simulink model "EVdemo_6"  (R2013b)
settings: Solver=FixedStepDiscrete  SolverMode=SingleTasking  StartTime=0.0  StopTime=650  FixedStep=4e-5  MaxStep=1e-5  RelTol=1e-3
InitFcn:
  | %EV_Param_Update
  | % update the number of strings (discretized)
  | numStrings = round(Opti_numStrings);
  | %disp(['Number of strings: ' num2str(numStrings)])
  | % update the effective capacity based on the number of strings
  | EV_Param.Battery_Det.Rated_Capacity = 28.5*numStrings; %A*hr
  | EV_Param.Battery_Det.DP = 1.5*fliplr([1500 1500 1600 1450 1325 1125 925 675 425 175 ])./8*EV_Param.Battery_Det.Rated_Capacity; % 8 comes from the 8Ahr rated batter data used (normalize and rescale to the rated capacity
  | EV_Param.Battery_Det.CP = fliplr([25 100 200 250 375 550 750 950 1125 1150])./8*EV_Param.Battery_Det.Rated_Capacity;
  | 
  | % update the number of cells in a string (discretized)
  | numSeriesCells = round(Opti_numSeriesCells);
  | %disp(['Number of cells in a string: ' num2str(numSeriesCells)])
  | % update the nominal string volage and charge deficit
  | EV_Param.Battery_Det.Nominal_Voltage = numSeriesCells*cellVolts;
  | BatteryParams(1).Qe_init = 0;%EV_Param.Battery_Det.Rated_Capacity*(1-EV_Param.Battery_Det.Initial_SOC/100); %Ampere*hours
  | 
  | % update the total number of cells, battery pack mass and total vehicle
  | % mass
  | total_cells = numSeriesCells*numStrings;
  | %disp(['Total Number of cells: ' num2str(total_cells)])
  | EV_Param.BatteryMass = BatteryParams(1).cell_mass*total_cells;
  | %disp(['Total Battery Pack Mass: ' num2str(EV_Param.BatteryMass)])
  | EV_Param.Vehicle.Mass = 1300+EV_Param.BatteryMass;
  | 
  | % update the driveline gear ratio
  | EV_Param.Vehicle.Engine_Vehicle_Gear_Ratio = Opti_Vehicle_Gear_Ratio;
  | %disp(['Driveline gear ratio: ' num2str(Opti_Vehicle_Gear_Ratio)])
StartFcn:
  | %tic;
StopFcn:
  | %toc;
  | %disp([Final SOC: ' num2str(SOC_final)])
  | %disp([Final Vehicle Error: ' num2str(normed_SQE_final)])
model workspace (MAT data in the model file):
  MCOS : class17 (value not decoded)
  MCOS : class17 (value not decoded)
values from neighbouring files (symbols this model uses):
  Drive_Cycle_Num = 8    [startDemo.m]
undefined symbols (not defined in the file or in its folder): Acc_Cmd, BatteryParams, Brake_Set, cell_area, ctrlConst, current_phase_a, Dec_Cmd, direct_current, DiscIntNeverNeededParam, electromagnetic_torque, HEV_Param, Ion, Kt_Temps, Lithium, Mech_Power_kW, Opti_numSeriesCells, Opti_numStrings, Opti_Vehicle_Gear_Ratio, paramVelocityI, paramVelocityP, paramVelocityPICurrentSat, pmsm, quadrature_current, RLoadLoss, rotor_velocity, sigbuilder_block, Ts, Veh_Spd_Ref
libraries: fl_lib x306, nesl_utility x100, LeadAcidBattery_lib x60, simulink x23, powerlib x16, sdl_lib x7, elec_lib x4, electricdrivelib x2, checkpacklib x2, CustomDriveline_lib x2, LiBatteryBlocks x1, Capacitors_lib x1
(part 5 of 7)

== system EVdemo_6/Battery/Cells/Battery cell8 ==
  C1 : LeadAcidBattery_lib/Main Branch Capacitance, C1  Tau1=HEV_Param.Battery_Cell.Tau1 s  Cmin=1e-5 F  i_Log=off  Q_Log=off  LocalVarNames=|i|v|Q  LocalVarDescs=|Current through variable|Voltage across variable|Charge variable  LocalVarLogging=[0 0 0]
  Diode : fl_lib/Electrical/Electrical Elements/Diode  Vf=0.6 V  Ron=0.3 Ohm  Goff=1e-08 1/Ohm  i_Log=off  v_Log=off  LocalVarNames=|current|voltage|power  LocalVarDescs=|Diode current (A)|Voltage across diode (V)|Power (W)  LocalVarLogging=[0 0 0]
  Ep : fl_lib/Electrical/Electrical Sources/DC Voltage Source  v0=HEV_Param.Battery_Cell.Ep V  i_Log=off  v_Log=off  LocalVarNames=|current|voltage|power  LocalVarDescs=|Current (A)|Voltage (V)|Power (W)  LocalVarLogging=[0 0 0]
  Main Branch Voltage Source (Em) : LeadAcidBattery_lib/Main Branch Voltage Source, Em  Em0=HEV_Param.Battery_Cell.Emo V  Ke=HEV_Param.Battery_Cell.Ke V/K  Kc=HEV_Param.Battery_Cell.Kc  C0=HEV_Param.Battery_Cell.Costar s*A  Istar=HEV_Param.Battery_Cell.Istar A  delta=HEV_Param.Battery_Cell.delta  Tau1=HEV_Param.Battery_Cell.Tau1 s  Qinit=HEV_Param.Battery_Cell.Qe_init s*A  i_Log=off  Iavg_Log=off  Qe_Log=off  LocalVarNames=|i|v|cap_u|cap_t|Q|Iavg  LocalVarDescs=|Current through variable|Voltage across variable|usable battery capacity|total battery capacity|battery charge|average current given by (I/(Ts+1))  LocalVarLogging=[0 0 0 0 0 0]
  R0 : LeadAcidBattery_lib/Terminal Resistance, R0  R00=HEV_Param.Battery_Cell.Roo Ohm  A0=HEV_Param.Battery_Cell.Ao  i_Log=off  LocalVarNames=|i|v  LocalVarDescs=|Current through variable|Voltage across variable  LocalVarLogging=[0 0]
  R1 : LeadAcidBattery_lib/Main Branch Resistance, R1  R10=HEV_Param.Battery_Cell.R10 Ohm  DOC_min=1e-006  i_Log=off  LocalVarNames=|i|v  LocalVarDescs=|Current through variable|Voltage across variable  LocalVarLogging=[0 0]
  R2 : LeadAcidBattery_lib/Main Branch Resistance, R2  R20=HEV_Param.Battery_Cell.R20 Ohm  A21=HEV_Param.Battery_Cell.A21  A22=HEV_Param.Battery_Cell.A22  Istar=HEV_Param.Battery_Cell.Istar A  i_Log=off  LocalVarNames=|i|v  LocalVarDescs=|Current through variable|Voltage across variable  LocalVarLogging=[0 0]
  Rp : LeadAcidBattery_lib/Parasitic Branch Resistance, Rp  Gp0=HEV_Param.Battery_Cell.Gpo 1/Ohm  Vp0=HEV_Param.Battery_Cell.Vpo V  Ap=HEV_Param.Battery_Cell.Ap  Tf=HEV_Param.Battery_Cell.theta_f C  i_Log=off  LocalVarNames=|i|v|Vavg  LocalVarDescs=|Current through variable|Voltage across variable|average voltage given by (V/(Ts+1))  LocalVarLogging=[0 0 0]
  Thermal Model : Subsystem
  H : PMIOPort  Tag=PMCPort  Port=1  Side=Left
  + : PMIOPort  Tag=PMCPort  Port=2  Side=Left
  - : PMIOPort  Tag=PMCPort  Port=3  Side=Right
  connections:
  Diode/LConn1 -- R0/RConn1 -- R2/LConn2
  R2/RConn2 -- Thermal Model/LConn1
  -/RConn1 -- Ep/RConn1 -- Main Branch Voltage Source (Em)/RConn1
  Thermal Model/RConn1 -- Main Branch Voltage Source (Em)/RConn3
  Diode/RConn1 -- Rp/LConn1
  Ep/LConn1 -- Rp/RConn2
  Thermal Model/LConn2 -- H/RConn1
  R0/LConn1 -- R2/LConn1 -- Main Branch Voltage Source (Em)/LConn1
  R1/LConn2 -- C1/LConn1
  R1/LConn1 -- C1/LConn2 -- R2/RConn1
  Main Branch Voltage Source (Em)/LConn3 -- C1/RConn1 -- R1/RConn2
  R1/RConn1 -- Main Branch Voltage Source (Em)/LConn2
  R0/LConn2 -- +/RConn1
  Thermal Model/RConn2 -- Main Branch Voltage Source (Em)/RConn2 -- Rp/RConn1

== system EVdemo_6/Battery/Cells/Battery cell9 ==
  C1 : LeadAcidBattery_lib/Main Branch Capacitance, C1  Tau1=HEV_Param.Battery_Cell.Tau1 s  Cmin=1e-5 F  i_Log=off  Q_Log=off  LocalVarNames=|i|v|Q  LocalVarDescs=|Current through variable|Voltage across variable|Charge variable  LocalVarLogging=[0 0 0]
  Diode : fl_lib/Electrical/Electrical Elements/Diode  Vf=0.6 V  Ron=0.3 Ohm  Goff=1e-08 1/Ohm  i_Log=off  v_Log=off  LocalVarNames=|current|voltage|power  LocalVarDescs=|Diode current (A)|Voltage across diode (V)|Power (W)  LocalVarLogging=[0 0 0]
  Ep : fl_lib/Electrical/Electrical Sources/DC Voltage Source  v0=HEV_Param.Battery_Cell.Ep V  i_Log=off  v_Log=off  LocalVarNames=|current|voltage|power  LocalVarDescs=|Current (A)|Voltage (V)|Power (W)  LocalVarLogging=[0 0 0]
  Main Branch Voltage Source (Em) : LeadAcidBattery_lib/Main Branch Voltage Source, Em  Em0=HEV_Param.Battery_Cell.Emo V  Ke=HEV_Param.Battery_Cell.Ke V/K  Kc=HEV_Param.Battery_Cell.Kc  C0=HEV_Param.Battery_Cell.Costar s*A  Istar=HEV_Param.Battery_Cell.Istar A  delta=HEV_Param.Battery_Cell.delta  Tau1=HEV_Param.Battery_Cell.Tau1 s  Qinit=HEV_Param.Battery_Cell.Qe_init s*A  i_Log=off  Iavg_Log=off  Qe_Log=off  LocalVarNames=|i|v|cap_u|cap_t|Q|Iavg  LocalVarDescs=|Current through variable|Voltage across variable|usable battery capacity|total battery capacity|battery charge|average current given by (I/(Ts+1))  LocalVarLogging=[0 0 0 0 0 0]
  R0 : LeadAcidBattery_lib/Terminal Resistance, R0  R00=HEV_Param.Battery_Cell.Roo Ohm  A0=HEV_Param.Battery_Cell.Ao  i_Log=off  LocalVarNames=|i|v  LocalVarDescs=|Current through variable|Voltage across variable  LocalVarLogging=[0 0]
  R1 : LeadAcidBattery_lib/Main Branch Resistance, R1  R10=HEV_Param.Battery_Cell.R10 Ohm  DOC_min=1e-006  i_Log=off  LocalVarNames=|i|v  LocalVarDescs=|Current through variable|Voltage across variable  LocalVarLogging=[0 0]
  R2 : LeadAcidBattery_lib/Main Branch Resistance, R2  R20=HEV_Param.Battery_Cell.R20 Ohm  A21=HEV_Param.Battery_Cell.A21  A22=HEV_Param.Battery_Cell.A22  Istar=HEV_Param.Battery_Cell.Istar A  i_Log=off  LocalVarNames=|i|v  LocalVarDescs=|Current through variable|Voltage across variable  LocalVarLogging=[0 0]
  Rp : LeadAcidBattery_lib/Parasitic Branch Resistance, Rp  Gp0=HEV_Param.Battery_Cell.Gpo 1/Ohm  Vp0=HEV_Param.Battery_Cell.Vpo V  Ap=HEV_Param.Battery_Cell.Ap  Tf=HEV_Param.Battery_Cell.theta_f C  i_Log=off  LocalVarNames=|i|v|Vavg  LocalVarDescs=|Current through variable|Voltage across variable|average voltage given by (V/(Ts+1))  LocalVarLogging=[0 0 0]
  Thermal Model : Subsystem
  H : PMIOPort  Tag=PMCPort  Port=1  Side=Left
  + : PMIOPort  Tag=PMCPort  Port=2  Side=Left
  - : PMIOPort  Tag=PMCPort  Port=3  Side=Right
  connections:
  Diode/LConn1 -- R0/RConn1 -- R2/LConn2
  R2/RConn2 -- Thermal Model/LConn1
  -/RConn1 -- Ep/RConn1 -- Main Branch Voltage Source (Em)/RConn1
  Thermal Model/RConn1 -- Main Branch Voltage Source (Em)/RConn3
  Diode/RConn1 -- Rp/LConn1
  Ep/LConn1 -- Rp/RConn2
  Thermal Model/LConn2 -- H/RConn1
  R0/LConn1 -- R2/LConn1 -- Main Branch Voltage Source (Em)/LConn1
  R1/LConn2 -- C1/LConn1
  R1/LConn1 -- C1/LConn2 -- R2/RConn1
  Main Branch Voltage Source (Em)/LConn3 -- C1/RConn1 -- R1/RConn2
  R1/RConn1 -- Main Branch Voltage Source (Em)/LConn2
  R0/LConn2 -- +/RConn1
  Thermal Model/RConn2 -- Main Branch Voltage Source (Em)/RConn2 -- Rp/RConn1

== system EVdemo_6/Battery/Cells/Intf ==
  Controlled Voltage Source : fl_lib/Electrical/Electrical Sources/Controlled Voltage Source  i_Log=off  v_Log=off  LocalVarNames=|i|v  LocalVarDescs=|i|v  LocalVarLogging=[0 0]
  Controlled Current Source : fl_lib/Electrical/Electrical Sources/Controlled Current Source  i_Log=off  v_Log=off  LocalVarNames=|i|v  LocalVarDescs=|i|v  LocalVarLogging=[0 0]
  Current Sensor : fl_lib/Electrical/Electrical Sensors/Current Sensor  i1_Log=off  v1_Log=off  LocalVarNames=|i1|v1  LocalVarDescs=|i1|v1  LocalVarLogging=[0 0]
  PS-Simulink Converter : nesl_utility/PS-Simulink Converter  PhysicalDomain=network_engine_domain  SubClassName=ps_output  LeftPortType=input  RightPortType=output  PseudoPeriodic=off  Frequencies=[]  Unit=A  AffineConversion=off
  PS-Simulink Converter1 : nesl_utility/PS-Simulink Converter  PhysicalDomain=network_engine_domain  SubClassName=ps_output  LeftPortType=input  RightPortType=output  PseudoPeriodic=off  Frequencies=[]  Unit=V  AffineConversion=off
  Simulink-PS Converter : nesl_utility/Simulink-PS Converter  PhysicalDomain=network_engine_domain  SubClassName=ps_input  LeftPortType=input  RightPortType=output  PseudoPeriodic=off  Frequencies=[]  NoiseDistribution=none  NoiseParameters=[]  Unit=V  AffineConversion=off  InputFiltering=off  SimscapeFilterOrder=1  InputFilterTimeConstant=.001  UdotUserProvided=0
  Simulink-PS Converter1 : nesl_utility/Simulink-PS Converter  PhysicalDomain=network_engine_domain  SubClassName=ps_input  LeftPortType=input  RightPortType=output  PseudoPeriodic=off  Frequencies=[]  NoiseDistribution=none  NoiseParameters=[]  Unit=A  AffineConversion=off  InputFiltering=off  SimscapeFilterOrder=1  InputFilterTimeConstant=.001  UdotUserProvided=0
  Transfer Fcn : TransferFcn  Denominator=[1/T 1]
  Voltage Sensor : fl_lib/Electrical/Electrical Sensors/Voltage Sensor  i1_Log=off  v1_Log=off  LocalVarNames=|i1|v1  LocalVarDescs=|i1|v1  LocalVarLogging=[0 0]
  + SPS : PMIOPort  Port=1  Side=Left
  - SPS : PMIOPort  Port=2  Side=Left
  SSC + : PMIOPort  Port=3  Side=Right
  SSC - : PMIOPort  Port=4  Side=Right
  wires:
  PS-Simulink Converter1/1 -> Transfer Fcn/1
  Transfer Fcn/1 -> Simulink-PS Converter/1
  PS-Simulink Converter/1 -> Simulink-PS Converter1/1
  connections:
  Controlled Current Source/RConn1 -- Simulink-PS Converter1/RConn1
  PS-Simulink Converter1/LConn1 -- Voltage Sensor/RConn1
  Voltage Sensor/LConn1 -- + SPS/RConn1 -- Controlled Current Source/LConn1
  Current Sensor/RConn2 -- SSC -/RConn1
  Voltage Sensor/RConn2 -- - SPS/RConn1 -- Controlled Current Source/RConn2
  Current Sensor/RConn1 -- PS-Simulink Converter/LConn1
  Simulink-PS Converter/RConn1 -- Controlled Voltage Source/RConn1
  Current Sensor/LConn1 -- Controlled Voltage Source/RConn2
  Controlled Voltage Source/LConn1 -- SSC +/RConn1

== system EVdemo_6/Battery/Cells/Measurements ==
  Bus Creator : BusCreator
  Calc Pct : Gain  Gain=1/HEV_Param.Battery_Sys.Maximum_Capacity*100
  Calculate battery power & charge : Subsystem
  PS-Simulink Converter1 : nesl_utility/PS-Simulink Converter  PhysicalDomain=network_engine_domain  SubClassName=ps_output  LeftPortType=input  RightPortType=output  PseudoPeriodic=off  Frequencies=[]  Unit=V  AffineConversion=off
  PS-Simulink Converter2 : nesl_utility/PS-Simulink Converter  PhysicalDomain=network_engine_domain  SubClassName=ps_output  LeftPortType=input  RightPortType=output  PseudoPeriodic=off  Frequencies=[]  Unit=A  AffineConversion=off
  VBatt : PMIOPort  Port=1  Side=Left
  IBatt : PMIOPort  Port=2  Side=Left
  Batt_Ah : Outport
  Batt_Meas : Outport  Port=2
  tag scope: Batt_Measures=global
  wires:
  Bus Creator/1 -> Batt_Meas/1, [Batt_Measures]
  PS-Simulink Converter2/1 -> Bus Creator/4  "Current (A)"
  PS-Simulink Converter1/1 -> Bus Creator/3  "Voltage (V)"
  Calc Pct/1 -> Bus Creator/2  "SOC (%)"
  Calculate battery power & charge/1(Ah) -> Batt_Ah/1, Calc Pct/1, Bus Creator/1  "Batt_Ah"
  connections:
  PS-Simulink Converter2/LConn1 -- IBatt/RConn1 -- Calculate battery power & charge/LConn2
  PS-Simulink Converter1/LConn1 -- VBatt/RConn1 -- Calculate battery power & charge/LConn1

== system EVdemo_6/Battery/Cells/Subsystem ==
  Voltage Sensor1 : fl_lib/Electrical/Electrical Sensors/Voltage Sensor  i1_Log=off  v1_Log=off  LocalVarNames=|i1|v1  LocalVarDescs=|i1|v1  LocalVarLogging=[]
  Conn1 : PMIOPort  Port=1  Side=Right
  Conn2 : PMIOPort  Port=2  Side=Left
  Conn3 : PMIOPort  Port=3  Side=Right
  connections:
  Conn3/RConn1 -- Voltage Sensor1/RConn2
  Conn2/RConn1 -- Voltage Sensor1/LConn1
  Conn1/RConn1 -- Voltage Sensor1/RConn1

== system EVdemo_6/Battery/Cells/Subsystem1 ==
  Current Sensor : fl_lib/Electrical/Electrical Sensors/Current Sensor  i1_Log=off  v1_Log=off  LocalVarNames=|i1|v1  LocalVarDescs=|i1|v1  LocalVarLogging=[]
  Conn1 : PMIOPort  Port=1  Side=Left
  Conn3 : PMIOPort  Port=2  Side=Right
  Conn2 : PMIOPort  Port=3  Side=Right
  connections:
  Conn3/RConn1 -- Current Sensor/RConn2
  Conn2/RConn1 -- Current Sensor/RConn1
  Conn1/RConn1 -- Current Sensor/LConn1

== system EVdemo_6/Battery/Generic/Measurements ==
  Bus Creator : BusCreator
  Calc Pct : Gain  Gain=1/HEV_Param.Battery_Sys.Maximum_Capacity*100
  Calculate battery power & charge : Subsystem
  PS-Simulink Converter1 : nesl_utility/PS-Simulink Converter  PhysicalDomain=network_engine_domain  SubClassName=ps_output  LeftPortType=input  RightPortType=output  PseudoPeriodic=off  Frequencies=[]  Unit=V  AffineConversion=off
  PS-Simulink Converter2 : nesl_utility/PS-Simulink Converter  PhysicalDomain=network_engine_domain  SubClassName=ps_output  LeftPortType=input  RightPortType=output  PseudoPeriodic=off  Frequencies=[]  Unit=A  AffineConversion=off
  VBatt : PMIOPort  Port=1  Side=Left
  IBatt : PMIOPort  Port=2  Side=Left
  Batt_Ah : Outport
  Batt_Meas : Outport  Port=2
  tag scope: Batt_Measures=global
  wires:
  Calculate battery power & charge/1(Ah) -> Bus Creator/1, Calc Pct/1, Batt_Ah/1  "Batt_Ah"
  Calc Pct/1 -> Bus Creator/2  "SOC (%)"
  PS-Simulink Converter1/1 -> Bus Creator/3  "Voltage (V)"
  PS-Simulink Converter2/1 -> Bus Creator/4  "Current (A)"
  Bus Creator/1 -> [Batt_Measures], Batt_Meas/1
  connections:
  Calculate battery power & charge/LConn1 -- VBatt/RConn1 -- PS-Simulink Converter1/LConn1
  Calculate battery power & charge/LConn2 -- IBatt/RConn1 -- PS-Simulink Converter2/LConn1

== system EVdemo_6/Battery/Generic1/Measurements ==
  Bus Creator : BusCreator
  Calc Pct : Gain  Gain=1/HEV_Param.Battery_Sys.Maximum_Capacity*100
  Calculate battery power & charge : Subsystem
  PS-Simulink Converter1 : nesl_utility/PS-Simulink Converter  PhysicalDomain=network_engine_domain  SubClassName=ps_output  LeftPortType=input  RightPortType=output  PseudoPeriodic=off  Frequencies=[]  Unit=V  AffineConversion=off
  PS-Simulink Converter2 : nesl_utility/PS-Simulink Converter  PhysicalDomain=network_engine_domain  SubClassName=ps_output  LeftPortType=input  RightPortType=output  PseudoPeriodic=off  Frequencies=[]  Unit=A  AffineConversion=off
  VBatt : PMIOPort  Port=1  Side=Left
  IBatt : PMIOPort  Port=2  Side=Left
  Batt_Ah : Outport
  Batt_Meas : Outport  Port=2
  tag scope: Batt_Measures=global
  wires:
  Bus Creator/1 -> Batt_Meas/1, [Batt_Measures]
  PS-Simulink Converter2/1 -> Bus Creator/4  "Current (A)"
  PS-Simulink Converter1/1 -> Bus Creator/3  "Voltage (V)"
  Calc Pct/1 -> Bus Creator/2  "SOC (%)"
  Calculate battery power & charge/1(Ah) -> Batt_Ah/1, Calc Pct/1, Bus Creator/1  "Batt_Ah"
  connections:
  PS-Simulink Converter2/LConn1 -- IBatt/RConn1 -- Calculate battery power & charge/LConn2
  PS-Simulink Converter1/LConn1 -- VBatt/RConn1 -- Calculate battery power & charge/LConn1

== system EVdemo_6/Battery/Predefined/GF1 ==
  In1 : Inport
  SOC Offset : Subsystem
      mask Display: disp('A')
  Out1 : Outport
  tag scope: Batt_Measures=global
  wires:
  In1/1 -> SOC Offset/1(In1)
  SOC Offset/1(Out1) -> [Batt_Measures], Out1/1

== system EVdemo_6/Battery/Predefined/Intf ==
  Controlled Voltage Source : fl_lib/Electrical/Electrical Sources/Controlled Voltage Source  i_Log=off  v_Log=off  LocalVarNames=|i|v  LocalVarDescs=|i|v  LocalVarLogging=[0 0]
  Controlled Current Source : powerlib/Electrical Sources/Controlled Current Source  Initialize=on  Source_Type=AC  Amplitude=0  Phase=0  Frequency=0  Measurements=None
  Current Sensor : fl_lib/Electrical/Electrical Sensors/Current Sensor  i1_Log=off  v1_Log=off  LocalVarNames=|i1|v1  LocalVarDescs=|i1|v1  LocalVarLogging=[0 0]
  Current-Voltage Simscape Interface : powerlib/Interface Elements/Current-Voltage Simscape Interface  DFT=off  FMode=Low pass filter (continuous)  T=1e-6  Ts=50e-6  i0=0  v0=0  Sd=SimPowerSystems side  Measurements=off
  PS-Simulink Converter : nesl_utility/PS-Simulink Converter  PhysicalDomain=network_engine_domain  SubClassName=ps_output  LeftPortType=input  RightPortType=output  PseudoPeriodic=off  Frequencies=[]  Unit=A  AffineConversion=off
  Simulink-PS Converter : nesl_utility/Simulink-PS Converter  PhysicalDomain=network_engine_domain  SubClassName=ps_input  LeftPortType=input  RightPortType=output  PseudoPeriodic=off  Frequencies=[]  NoiseDistribution=none  NoiseParameters=[]  Unit=V  AffineConversion=off  InputFiltering=off  SimscapeFilterOrder=1  InputFilterTimeConstant=.001  UdotUserProvided=0
  Transfer Fcn : TransferFcn  Denominator=[1/T 1]
  Voltage Measurement : powerlib/Measurements/Voltage Measurement  PhasorSimulation=off  OutputType=Complex  PSBequivalent=0
  + SPS : PMIOPort  Port=1  Side=Left
  - SPS : PMIOPort  Port=2  Side=Left
  SSC + : PMIOPort  Port=3  Side=Right
  SSC - : PMIOPort  Port=4  Side=Right
  wires:
  PS-Simulink Converter/1 -> Controlled Current Source/1
  Voltage Measurement/1 -> Transfer Fcn/1
  Transfer Fcn/1 -> Simulink-PS Converter/1
  connections:
  Controlled Voltage Source/LConn1 -- SSC +/RConn1
  Current Sensor/LConn1 -- Controlled Voltage Source/RConn2
  Simulink-PS Converter/RConn1 -- Controlled Voltage Source/RConn1
  Current Sensor/RConn1 -- PS-Simulink Converter/LConn1
  Controlled Current Source/LConn1 -- Voltage Measurement/LConn2 -- - SPS/RConn1
  Current Sensor/RConn2 -- SSC -/RConn1
  Controlled Current Source/RConn1 -- + SPS/RConn1 -- Voltage Measurement/LConn1

== system EVdemo_6/Battery/RCGeneric/Measurements ==
  Bus Creator : BusCreator
  Calc Pct : Gain  Gain=1/HEV_Param.Battery_Sys.Maximum_Capacity*100
  Calculate battery power & charge : Subsystem
  PS-Simulink Converter1 : nesl_utility/PS-Simulink Converter  PhysicalDomain=network_engine_domain  SubClassName=ps_output  LeftPortType=input  RightPortType=output  PseudoPeriodic=off  Frequencies=[]  Unit=V  AffineConversion=off
  PS-Simulink Converter2 : nesl_utility/PS-Simulink Converter  PhysicalDomain=network_engine_domain  SubClassName=ps_output  LeftPortType=input  RightPortType=output  PseudoPeriodic=off  Frequencies=[]  Unit=A  AffineConversion=off
  VBatt : PMIOPort  Port=1  Side=Left
  IBatt : PMIOPort  Port=2  Side=Left
  Batt_Ah : Outport
  Batt_Meas : Outport  Port=2
  tag scope: Batt_Measures=global
  wires:
  Calculate battery power & charge/1(Ah) -> Bus Creator/1, Calc Pct/1, Batt_Ah/1  "Batt_Ah"
  Calc Pct/1 -> Bus Creator/2  "SOC (%)"
  PS-Simulink Converter1/1 -> Bus Creator/3  "Voltage (V)"
  PS-Simulink Converter2/1 -> Bus Creator/4  "Current (A)"
  Bus Creator/1 -> [Batt_Measures], Batt_Meas/1
  connections:
  Calculate battery power & charge/LConn1 -- VBatt/RConn1 -- PS-Simulink Converter1/LConn1
  Calculate battery power & charge/LConn2 -- IBatt/RConn1 -- PS-Simulink Converter2/LConn1

== system EVdemo_6/DCDC_Converter/Detailed DC//DC Converter/PWM ==
  Ref. : Inport
  Data Type Conversion : DataTypeConversion  SaturateOnIntegerOverflow=on  RndMeth=Zero
  Data Type Conversion1 : DataTypeConversion  SaturateOnIntegerOverflow=on  RndMeth=Zero
  Mux : Mux  Inputs=2
  NOT : Logic  Operator=NOT  Inputs=1  AllPortsSameDT=off  OutDataTypeStr=uint(8)
  Rate Transition : RateTransition
  Relational Operator : RelationalOperator  Operator=>
  Sawtooth generator : Subsystem
  Thermal Model : Subsystem  Commented=on
  Zero-Order Hold : ZeroOrderHold  SampleTime=Ts
  Pulses : Outport
  wires:
  Data Type Conversion1/1 -> Pulses/1
  Mux/1 -> Data Type Conversion1/1
  Ref./1 -> Thermal Model/1(IBus), Rate Transition/1
  Sawtooth generator/1(Out) -> Relational Operator/2
  Zero-Order Hold/1 -> Relational Operator/1
  Data Type Conversion/1 -> NOT/1, Mux/1
  Relational Operator/1 -> Data Type Conversion/1
  Rate Transition/1 -> Zero-Order Hold/1
  NOT/1 -> Mux/2

== system EVdemo_6/DCDC_Converter/Detailed DC//DC Converter/Subsystem ==
  PS-Simulink Converter1 : nesl_utility/PS-Simulink Converter  PhysicalDomain=network_engine_domain  SubClassName=ps_output  LeftPortType=input  RightPortType=output  PseudoPeriodic=off  Frequencies=[]  Unit=C  AffineConversion=on
  In : PMIOPort  Port=1  Side=Left
  Out : PMIOPort  Port=2  Side=Right
  tag scope: DCDC_Power_Loss=global
  wires:
  PS-Simulink Converter1/1 -> [DCDC_Power_Loss]
  connections:
  Out/RConn1 -- PS-Simulink Converter1/LConn1 -- In/RConn1

== system EVdemo_6/DCDC_Converter/Detailed DC//DC Converter/Subsystem1 ==
  IBus : Inport
  PToHeat : Gain  Gain=HEV_Param.DCDCConv.EPower2Heat  SaturateOnIntegerOverflow=on  OutDataTypeStr=Inherit: Same as input  ParamDataTypeStr=Inherit: Same as input
  Product : Product  RndMeth=Zero
  RLoss : Gain  Gain=HEV_Param.DCDCConv.Resistance_Losses  SaturateOnIntegerOverflow=on  OutDataTypeStr=Inherit: Same as input  ParamDataTypeStr=Inherit: Same as input
  Heat Flow : Outport
  wires:
  PToHeat/1 -> Heat Flow/1
  RLoss/1 -> PToHeat/1
  IBus/1 -> Product/2, Product/1
  Product/1 -> RLoss/1

== system EVdemo_6/DCDC_Converter/Detailed DC//DC Converter/Temperature Sensor ==
  Ideal Temperature Sensor : fl_lib/Thermal/Thermal Sensors/Ideal Temperature Sensor  Qs_Log=off  Ts_Log=off  LocalVarNames=|Qs|Ts  LocalVarDescs=|Qs|Ts  LocalVarLogging=[]
  PS-Simulink Converter : nesl_utility/PS-Simulink Converter  PhysicalDomain=network_engine_domain  SubClassName=ps_output  LeftPortType=input  RightPortType=output  PseudoPeriodic=off  Frequencies=[]  Unit=C  AffineConversion=on
  Rate Transition5 : RateTransition  OutPortSampleTime=.01
  Thermal Reference : fl_lib/Thermal/Thermal Elements/Thermal Reference  Q_Log=off  LocalVarNames=|Q  LocalVarDescs=|Q  LocalVarLogging=[]
  Conn2 : PMIOPort  Port=1  Side=Left
  tag scope: DCDC_SYS=global
  wires:
  PS-Simulink Converter/1 -> Rate Transition5/1  "DCDC_Temp"
  Rate Transition5/1 -> [DCDC_SYS]
  connections:
  Conn2/RConn1 -- Ideal Temperature Sensor/LConn1
  Thermal Reference/LConn1 -- Ideal Temperature Sensor/RConn1
  PS-Simulink Converter/LConn1 -- Ideal Temperature Sensor/RConn2

== system EVdemo_6/DCDC_Converter/Detailed DC//DC Converter/Voltage Controller ==
  Uref : Inport
  UBus : Inport  Port=2
  Clock1 : Clock
  Compare To Constant1 : simulink/Logic and Bit Operations/Compare To Constant  relop=>  const=0.01  OutDataTypeStr=uint8  ZeroCross=off
  Ctrl sat. : Saturate  UpperLimit=0.95  LowerLimit=-0.95
  Discrete-Time Integrator : DiscreteIntegrator  IntegratorMethod=Integration: Trapezoidal  SampleTime=Ts  LimitOutput=on  UpperSaturationLimit=1  LowerSaturationLimit=-1  ICPrevOutput=DiscIntNeverNeededParam  ICPrevScaledInput=DiscIntNeverNeededParam
  Integral gain : Gain  Gain=Ki  SaturateOnIntegerOverflow=on  OutDataTypeStr=Inherit: Same as input  ParamDataTypeStr=Inherit: Same as input
  Product1 : Product  RndMeth=Zero
  Proportional gain : Gain  Gain=Kp  SaturateOnIntegerOverflow=on  OutDataTypeStr=Inherit: Same as input  ParamDataTypeStr=Inherit: Same as input
  Sum1 : Sum  Inputs=+-  SaturateOnIntegerOverflow=on  InputSameDT=on  OutDataTypeStr=Inherit: Same as first input
  Sum2 : Sum  SaturateOnIntegerOverflow=on  InputSameDT=on  OutDataTypeStr=Inherit: Same as first input
  Transfer Fcn : TransferFcn  Denominator=[.0001 1]
  Zero-Order Hold1 : ZeroOrderHold  SampleTime=Ts
  Ec : Outport  InitialOutput=0
  wires:
  Uref/1 -> Sum1/2
  Transfer Fcn/1 -> Sum1/1
  Zero-Order Hold1/1 -> Transfer Fcn/1
  Product1/1 -> Proportional gain/1, Integral gain/1
  Compare To Constant1/1 -> Product1/2
  Clock1/1 -> Compare To Constant1/1
  Sum1/1 -> Product1/1
  Ctrl sat./1 -> Ec/1
  Proportional gain/1 -> Sum2/1
  Integral gain/1 -> Discrete-Time Integrator/1
  UBus/1 -> Zero-Order Hold1/1
  Discrete-Time Integrator/1 -> Sum2/2
  Sum2/1 -> Ctrl sat./1

== system EVdemo_6/DCDC_Converter/System DC-DC Converter/Calcuate Input Current Pout+PLoss = Pin2 ==
  note: Total Power
  note: Power Output
  Input^2 : fl_lib/Physical Signals/Functions/PS Math Function  fcn_choice=7  LocalVarLogging=[]
  No Div By 0 : fl_lib/Physical Signals/Nonlinear Operators/PS Max  LocalVarLogging=[]
  PS Add : fl_lib/Physical Signals/Functions/PS Add  LocalVarLogging=[]
  PS Constant : fl_lib/Physical Signals/Sources/PS Constant  constant=EV_Param.DCDCConv.MinVin  LocalVarLogging=[]
  PS Divide : fl_lib/Physical Signals/Functions/PS Divide  LocalVarLogging=[]
  PS Product : fl_lib/Physical Signals/Functions/PS Product  LocalVarLogging=[]
  RLoadLoss : fl_lib/Physical Signals/Functions/PS Gain  gain=RLoadLoss  LocalVarLogging=[]
  V_In : PMIOPort  Port=1  Side=Left
  Iout : PMIOPort  Port=2  Side=Left
  Vout : PMIOPort  Port=3  Side=Left
  I_Input : PMIOPort  Port=4  Side=Right
  P Loss : PMIOPort  Port=5  Side=Right
  connections:
  PS Add/RConn1 -- PS Divide/LConn1
  No Div By 0/RConn1 -- PS Divide/LConn2
  V_In/RConn1 -- No Div By 0/LConn2
  No Div By 0/LConn1 -- PS Constant/RConn1
  P Loss/RConn1 -- RLoadLoss/RConn1 -- PS Add/LConn1
  PS Add/LConn2 -- PS Product/RConn1
  RLoadLoss/LConn1 -- Input^2/RConn1
  Iout/RConn1 -- PS Product/LConn1 -- Input^2/LConn1
  Vout/RConn1 -- PS Product/LConn2
  I_Input/RConn1 -- PS Divide/RConn1

== system EVdemo_6/DCDC_Converter/System DC-DC Converter/Control Bus Voltage ==
  V_fdbk : Inport
  Bus_Control : Subsystem
      mask Display:
      | disp('PI(z)')
      | port_label('input',1, 'Error');
      | port_label('output',1, 'V_cmd');
  Constant : Constant  Value=Vout
  Data Type Conversion1 : DataTypeConversion  OutDataTypeStr=double
  Data Type Conversion3 : DataTypeConversion  OutDataTypeStr=DT_PRECISION_LO
  Error Sum : Sum  Inputs=+-|  OutDataTypeStr=DT_PRECISION_LO
      settings: AttributesFormatString=-----------------------------\nMin = %<OutMin>\nMax = %<OutMax>
  Rate Transition : RateTransition  X0=650
  Rate Transition1 : RateTransition  X0=650
  Rate Transition3 : RateTransition  X0=650
  Unit Delay : UnitDelay  InitialCondition=650  SampleTime=-1
  V_satcmd : Outport
  wires:
  V_fdbk/1 -> Data Type Conversion3/1
  Rate Transition1/1 -> Unit Delay/1
  Constant/1 -> Rate Transition/1
  Unit Delay/1 -> Error Sum/2
  Rate Transition/1 -> Error Sum/1
  Bus_Control/1(V_Out) -> Rate Transition3/1
  Data Type Conversion3/1 -> Rate Transition1/1
  Data Type Conversion1/1 -> V_satcmd/1
  Rate Transition3/1 -> Data Type Conversion1/1
  Error Sum/1 -> Bus_Control/1(Err)

== system EVdemo_6/DCDC_Converter/System DC-DC Converter/Current Sensor2 ==
  Current Sensor : fl_lib/Electrical/Electrical Sensors/Current Sensor  i1_Log=off  v1_Log=off  LocalVarNames=|i1|v1  LocalVarDescs=|i1|v1  LocalVarLogging=[0 0]
  PS-Simulink Converter : nesl_utility/PS-Simulink Converter  PhysicalDomain=network_engine_domain  SubClassName=ps_output  LeftPortType=input  RightPortType=output  PseudoPeriodic=off  Frequencies=[]  Unit=1  AffineConversion=off
  I : PMIOPort  Port=1  Side=Right
  + : PMIOPort  Port=2  Side=Left
  - : PMIOPort  Port=3  Side=Right
  tag scope: I_out=global
  wires:
  PS-Simulink Converter/1 -> [I_out]
  connections:
  -/RConn1 -- Current Sensor/RConn2
  +/RConn1 -- Current Sensor/LConn1
  PS-Simulink Converter/LConn1 -- I/RConn1 -- Current Sensor/RConn1

== system EVdemo_6/DCDC_Converter/System DC-DC Converter/Subsystem ==
  PS-Simulink Converter1 : nesl_utility/PS-Simulink Converter  PhysicalDomain=network_engine_domain  SubClassName=ps_output  LeftPortType=input  RightPortType=output  PseudoPeriodic=off  Frequencies=[]  Unit=C  AffineConversion=on
  In : PMIOPort  Port=1  Side=Left
  Out : PMIOPort  Port=2  Side=Right
  tag scope: DCDC_Power_Loss=global
  wires:
  PS-Simulink Converter1/1 -> [DCDC_Power_Loss]
  connections:
  Out/RConn1 -- PS-Simulink Converter1/LConn1 -- In/RConn1

== system EVdemo_6/DCDC_Converter/System DC-DC Converter/Temperature Sensor ==
  Ideal Temperature Sensor : fl_lib/Thermal/Thermal Sensors/Ideal Temperature Sensor  Qs_Log=off  Ts_Log=off  LocalVarNames=|Qs|Ts  LocalVarDescs=|Qs|Ts  LocalVarLogging=[]
  PS-Simulink Converter : nesl_utility/PS-Simulink Converter  PhysicalDomain=network_engine_domain  SubClassName=ps_output  LeftPortType=input  RightPortType=output  PseudoPeriodic=off  Frequencies=[]  Unit=C  AffineConversion=on
  Terminator : Terminator
  Thermal Reference : fl_lib/Thermal/Thermal Elements/Thermal Reference  Q_Log=off  LocalVarNames=|Q  LocalVarDescs=|Q  LocalVarLogging=[]
  Conn2 : PMIOPort  Port=1  Side=Left
  wires:
  PS-Simulink Converter/1 -> Terminator/1  "DCDC_Temp"
  connections:
  Conn2/RConn1 -- Ideal Temperature Sensor/LConn1
  Thermal Reference/LConn1 -- Ideal Temperature Sensor/RConn1
  PS-Simulink Converter/LConn1 -- Ideal Temperature Sensor/RConn2

== system EVdemo_6/DCDC_Converter/System DC-DC Converter/Voltage Sensor Bus2 ==
  PS-Simulink Converter : nesl_utility/PS-Simulink Converter  PhysicalDomain=network_engine_domain  SubClassName=ps_output  LeftPortType=input  RightPortType=output  PseudoPeriodic=off  Frequencies=[]  Unit=1  AffineConversion=off
  Voltage Sensor Out : fl_lib/Electrical/Electrical Sensors/Voltage Sensor  i1_Log=off  v1_Log=off  LocalVarNames=|i1|v1  LocalVarDescs=|i1|v1  LocalVarLogging=[0 0]
  + : PMIOPort  Port=1  Side=Left
  - : PMIOPort  Port=2  Side=Right
  V : PMIOPort  Port=3  Side=Right
  tag scope: V_out=global
  wires:
  PS-Simulink Converter/1 -> [V_out]
  connections:
  -/RConn1 -- Voltage Sensor Out/RConn2
  PS-Simulink Converter/LConn1 -- Voltage Sensor Out/RConn1 -- V/RConn1
  +/RConn1 -- Voltage Sensor Out/LConn1

== system EVdemo_6/DCDC_Converter/System DC-DC Converter/Voltage Sensor2 ==
  PS-Simulink Converter : nesl_utility/PS-Simulink Converter  PhysicalDomain=network_engine_domain  SubClassName=ps_output  LeftPortType=input  RightPortType=output  PseudoPeriodic=off  Frequencies=[]  Unit=1  AffineConversion=off
  Voltage Sensor In : fl_lib/Electrical/Electrical Sensors/Voltage Sensor  i1_Log=off  v1_Log=off  LocalVarNames=|i1|v1  LocalVarDescs=|i1|v1  LocalVarLogging=[0 0]
  + : PMIOPort  Port=1  Side=Left
  V : PMIOPort  Port=2  Side=Right
  - : PMIOPort  Port=3  Side=Right
  tag scope: V_in=global
  wires:
  PS-Simulink Converter/1 -> [V_in]
  connections:
  PS-Simulink Converter/LConn1 -- Voltage Sensor In/RConn1 -- V/RConn1
  -/RConn1 -- Voltage Sensor In/RConn2
  +/RConn1 -- Voltage Sensor In/LConn1

== system EVdemo_6/Drive & Motor/Detailed_Motor/Continuous To Discrete1 ==
  note: Continuous To Discrete
  System Inputs : Inport
  Motor Measurements : Inport  Port=2
  Bus Selector : BusSelector  OutputSignals=Motor_Spd_Ref_radps
  Bus Selector3 : BusSelector  OutputSignals=motor.rotor_velocity,motor.current_phase_a,motor.current_phase_b,motor.electrical_position
  Motor On Data Type Conversion{1..4} (4 alike) : DataTypeConversion
  Motor On Rate Transition{1..4} (4 alike) : RateTransition  Deterministic=off
  Mux : Mux  Inputs=2
  Command : Outport
  Rotor Velocity : Outport  Port=2
  Phase Currents : Outport  Port=3
  Electrical Position : Outport  Port=4
  wires:
  Motor Measurements/1 -> Bus Selector3/1
  System Inputs/1 -> Bus Selector/1
  Bus Selector/1 -> Motor On Data Type Conversion2/1  "<Motor_Spd_Ref_radps>"
  Motor On Data Type Conversion2/1 -> Motor On Rate Transition3/1
  Motor On Rate Transition3/1 -> Command/1  "data"
  Bus Selector3/3 -> Mux/2  "<current_phase_b>"
  Bus Selector3/2 -> Mux/1  "<current_phase_a>"
  Mux/1 -> Motor On Data Type Conversion3/1
  Bus Selector3/1 -> Motor On Data Type Conversion1/1  "<rotor_velocity>"
  Bus Selector3/4 -> Motor On Data Type Conversion4/1  "<electrical_position>"
  Motor On Data Type Conversion1/1 -> Motor On Rate Transition1/1
  Motor On Data Type Conversion3/1 -> Motor On Rate Transition2/1
  Motor On Data Type Conversion4/1 -> Motor On Rate Transition4/1
  Motor On Rate Transition1/1 -> Rotor Velocity/1
  Motor On Rate Transition2/1 -> Phase Currents/1
  Motor On Rate Transition4/1 -> Electrical Position/1

== system EVdemo_6/Drive & Motor/Detailed_Motor/Discrete To Continuous1 ==
  note: Discrete To Continuous
  V : Inport
  Motor On Data Type Conversion1 : DataTypeConversion
  Motor On Rate Transition1 : RateTransition  Integrity=off  Deterministic=off
  Motor Command : Outport
  wires:
  V/1 -> Motor On Data Type Conversion1/1
  Motor On Rate Transition1/1 -> Motor Command/1
  Motor On Data Type Conversion1/1 -> Motor On Rate Transition1/1

== system EVdemo_6/Drive & Motor/Detailed_Motor/Motor And Sensors ==
  note: Bridge & Motor
  Controller : Inport
  Bus Creator2 : BusCreator  Inputs=2
  Ctrl sat. : Saturate  UpperLimit=1  LowerLimit=-1
  Detailed 3-Phase Inverter : powerlib/Power Electronics/Universal Bridge  Arms=3  SnubberResistance=5000  SnubberCapacitance=inf  Device=IGBT / Diodes  Ron=1e-3  Lon=0  ForwardVoltages=[0.7,0.7]*0  ForwardVoltage=0  GTOparameters=[ 10e-6 , 20e-6 ]  IGBTparameters=[0,0]  Measurements=None  Measurements_2=None  converterType=Rectifier
  Gain : Gain  Gain=1/ctrlConst.VoltageMax
  Ideal Heat Flow Source : fl_lib/Thermal/Thermal Sources/Ideal Heat Flow Source  Q_Log=off  T_Log=off  LocalVarNames=|heat_flow|T_differential  LocalVarDescs=|Heat flow through the source (J/s)|Temperature differential across the source (K)  LocalVarLogging=[0 0]
  Input^2 : fl_lib/Physical Signals/Functions/PS Math Function  fcn_choice=7  LocalVarLogging=[]
  PMSM_50kW : Subsystem
      mask Display: image('TorqueSpeedEfficiency.jpg')
  PWM Generator : powerlib_extras/Control  Blocks/PWM Generator  GeneratorMode="3-arm  bridge (6 pulses)"  Fc=1/HEV_Param.DCDCConv.PWM_Carrier_TS  Internal=off  mIndex=0.4  Freq=60  Phase=0
  RLoadLoss : fl_lib/Physical Signals/Functions/PS Gain  gain=RLoadLoss  LocalVarLogging=[]
  Simulink-PS Converter : nesl_utility/Simulink-PS Converter  PhysicalDomain=network_engine_domain  SubClassName=ps_input  LeftPortType=input  RightPortType=output  PseudoPeriodic=off  Frequencies=[]  NoiseDistribution=none  NoiseParameters=[]  Unit=1  AffineConversion=off  InputFiltering=off  SimscapeFilterOrder=1  InputFilterTimeConstant=0.001  UdotUserProvided=1
  Temperature Sensor : Subsystem
      mask Display:
      | patch([294.730220921338;294.546109275896;293.995547435362;293.083837611228;291.819760067491;290.215488561913;288.286473106077;286.051291173329;283.531468787557;280.75127321581;277.737479261253;274.519111407178;271.127164295357;267.594304230703;263.954554586898;260.242968142701;256.495289504528;252.747610866356;249.036024422158;245.396274778353;241.8634147137;238.471467601878;235.253099747803;232.239305793246;229.459110221499;226.939287835727;224.704105902979;222.775090447143;221.170818941565;219.906741397828;218.995031573694;218.44446973316;218.260358087718;218.44446973316;218.995031573694;219.906741397828;221.170818941565;222.775090447143;224.704105902979;226.939287835727;229.459110221499;232.239305793247;235.253099747803;238.471467601878;241.8634147137;245.396274778353;249.036024422158;252.747610866356;256.495289504528;260.242968142701;263.954554586898;267.594304230703;271.127164295357;274.519111407178;277.737479261253;280.75127321581;283.531468787557;286.051291173329;288.286473106077;290.215488561913;291.819760067491;293.083837611228;293.995547435362;294.546109275896;294.730220921338;294.730220921338], [122.389574535191;118.641895897019;114.930309452821;111.290559809016;107.757699744363;104.365752632541;101.147384778466;98.1335908239095;95.3533952521624;92.8335728663899;90.598390933642;88.6693754778057;87.0651039722279;85.8010264284914;84.8893166043572;84.3387547638233;84.1546431183815;84.3387547638233;84.8893166043572;85.8010264284914;87.0651039722279;88.6693754778058;90.598390933642;92.83357286639;95.3533952521625;98.1335908239095;101.147384778466;104.365752632541;107.757699744363;111.290559809016;114.930309452821;118.641895897019;122.389574535191;126.137253173364;129.848839617561;133.488589261366;137.02144932602;140.413396437841;143.631764291917;146.645558246473;149.42575381822;151.945576203992;154.18075813674;156.109773592576;157.714045098154;158.978122641891;159.889832466025;160.440394306559;160.624505952001;160.440394306559;159.889832466025;158.978122641891;157.714045098154;156.109773592576;154.18075813674;151.945576203992;149.42575381822;146.645558246473;143.631764291917;140.413396437841;137.02144932602;133.488589261366;129.848839617561;126.137253173364;122.389574535191;122.389574535191], [0;0;0])
      | plot([294.730220921338;294.546109275896;293.995547435362;293.083837611228;291.819760067491;290.215488561913;288.286473106077;286.051291173329;283.531468787557;280.75127321581;277.737479261253;274.519111407178;271.127164295357;267.594304230703;263.954554586898;260.242968142701;256.495289504528;252.747610866356;249.036024422158;245.396274778353;241.8634147137;238.471467601878;235.253099747803;232.239305793246;229.459110221499;226.939287835727;224.704105902979;222.775090447143;221.170818941565;219.906741397828;218.995031573694;218.44446973316;218.260358087718;218.44446973316;218.995031573694;219.906741397828;221.170818941565;222.775090447143;224.704105902979;226.939287835727;229.459110221499;232.239305793247;235.253099747803;238.471467601878;241.8634147137;245.396274778353;249.036024422158;252.747610866356;256.495289504528;260.242968142701;263.954554586898;267.594304230703;271.127164295357;274.519111407178;277.737479261253;280.75127321581;283.531468787557;286.051291173329;288.286473106077;290.215488561913;291.819760067491;293.083837611228;293.995547435362;294.546109275896;294.730220921338;294.730220921338], [122.389574535191;118.641895897019;114.930309452821;111.290559809016;107.757699744363;104.365752632541;101.147384778466;98.1335908239095;95.3533952521624;92.8335728663899;90.598390933642;88.6693754778057;87.0651039722279;85.8010264284914;84.8893166043572;84.3387547638233;84.1546431183815;84.3387547638233;84.8893166043572;85.8010264284914;87.0651039722279;88.6693754778058;90.598390933642;92.83357286639;95.3533952521625;98.1335908239095;101.147384778466;104.365752632541;107.757699744363;111.290559809016;114.930309452821;118.641895897019;122.389574535191;126.137253173364;129.848839617561;133.488589261366;137.02144932602;140.413396437841;143.631764291917;146.645558246473;149.42575381822;151.945576203992;154.18075813674;156.109773592576;157.714045098154;158.978122641891;159.889832466025;160.440394306559;160.624505952001;160.440394306559;159.889832466025;158.978122641891;157.714045098154;156.109773592576;154.18075813674;151.945576203992;149.42575381822;146.645558246473;143.631764291917;140.413396437841;137.02144932602;133.488589261366;129.848839617561;126.137253173364;122.389574535191;122.389574535191])
      | plot([243.771309033036;263.613159768283;263.613159768283;243.771309033036;243.771309033036], [438.410416245461;438.410416245461;112.4371541664;112.4371541664;438.410416245461])
      | plot([510.219018906355;0;0;510.219018906355;510.219018906355], [509.274168871343;509.274168871343;0;0;509.274168871343])
      | ;
      | %color('red');
      | %port_label('LConn', 1,'A')
      | %port_label('RConn', 1,'B')
  Thermal Mass : fl_lib/Thermal/Thermal Elements/Thermal Mass  mass=EV_Param.DCDCConv.Thermal_Mass kg  sp_heat=EV_Param.DCDCConv.Specific_Heat J/kg/K  init_temp=EV_Param.DCDCConv.Initial_Temperature C  Q_Log=off  LocalVarNames=|heat_flow|temperature  LocalVarDescs=|Heat flow (J/s)|Mass temperature (K)  LocalVarLogging=[0 0]
  Thermal Ref : fl_lib/Thermal/Thermal Elements/Thermal Reference  Q_Log=off  LocalVarNames=|Q  LocalVarDescs=|Q  LocalVarLogging=[]
  Three-Phase V-I Measurement : powerlib/Measurements/Three-Phase V-I Measurement  VoltageMeasurement=phase-to-phase  SetLabelV=off  LabelV=Vabc  Vpu=off  VpuLL=off  CurrentMeasurement=yes  SetLabelI=off  LabelI=Iabc  Ipu=off  Pbase=100e6  Vbase=500e3  OutputType=Complex  PhasorSimulation=off  PSBequivalent=0
  Voltage-Current Simscape Interface : powerlib/Interface Elements/Voltage-Current Simscape Interface  DFT=off  Fmode=Unit delay (discrete)  T=1e-6  Ts=-1  i0=0  v0=0  Sd=SimPowerSystems side  Measurements=off
  + : PMIOPort  Port=1  Side=Left
  - : PMIOPort  Port=2  Side=Left
  R : PMIOPort  Port=3  Side=Right
  H : PMIOPort  Port=4  Side=Left
  Motor_Fdbk : Outport
  wires:
  Bus Creator2/1 -> Motor_Fdbk/1
  PMSM_50kW/1(M) -> Bus Creator2/2  "motor"
  Three-Phase V-I Measurement/1 -> Bus Creator2/1  "phase_voltage"
  PWM Generator/1 -> Detailed 3-Phase Inverter/1  "Pulses*"
  Controller/1 -> Gain/1
  Gain/1 -> Ctrl sat./1
  Three-Phase V-I Measurement/2 -> Simulink-PS Converter/1
  Ctrl sat./1 -> PWM Generator/1
  connections:
  PMSM_50kW/RConn1 -- R/RConn1
  Detailed 3-Phase Inverter/LConn1 -- Three-Phase V-I Measurement/LConn1
  Detailed 3-Phase Inverter/LConn3 -- Three-Phase V-I Measurement/LConn3
  Detailed 3-Phase Inverter/LConn2 -- Three-Phase V-I Measurement/LConn2
  Three-Phase V-I Measurement/RConn1 -- PMSM_50kW/LConn1
  Three-Phase V-I Measurement/RConn3 -- PMSM_50kW/LConn3
  Three-Phase V-I Measurement/RConn2 -- PMSM_50kW/LConn2
  +/RConn1 -- Voltage-Current Simscape Interface/RConn1
  -/RConn1 -- Voltage-Current Simscape Interface/RConn2
  Detailed 3-Phase Inverter/RConn2 -- Voltage-Current Simscape Interface/LConn2
  RLoadLoss/LConn1 -- Input^2/RConn1
  Simulink-PS Converter/RConn1 -- Input^2/LConn1
  H/RConn1 -- Ideal Heat Flow Source/LConn1 -- Temperature Sensor/LConn1 -- Thermal Mass/LConn1
  Thermal Ref/LConn1 -- Ideal Heat Flow Source/RConn2
  Ideal Heat Flow Source/RConn1 -- RLoadLoss/RConn1
  Voltage-Current Simscape Interface/LConn1 -- Detailed 3-Phase Inverter/RConn1

== system EVdemo_6/Drive & Motor/Detailed_Motor/ZZZ_Background_Box ==

== system EVdemo_6/Drive & Motor/System_Motor/Continuous To Discrete1 ==
  note: Continuous To Discrete
  System Inputs : Inport
  Motor Measurements : Inport  Port=2
  Bus Selector : BusSelector  OutputSignals=Motor_Spd_Ref_radps,Motor_Limits.Motor_T_Lim,Motor_Limits.Regen_T_Lim
  Bus Selector3 : BusSelector  OutputSignals=Motor_Fdbk.rotor_velocity
  Motor On Data Type Conversion1 : DataTypeConversion
  Motor On Rate Transition{1..4} (4 alike) : RateTransition  Deterministic=off  OutPortSampleTime=ctrlConst.Ts
  Command : Outport
  Command1 : Outport  Port=2
  Command2 : Outport  Port=3
  Rotor Velocity : Outport  Port=4
  wires:
  Motor Measurements/1 -> Bus Selector3/1
  System Inputs/1 -> Bus Selector/1
  Bus Selector/1 -> Motor On Rate Transition3/1  "<Motor_Spd_Ref_radps>"
  Motor On Rate Transition3/1 -> Command/1  "data"
  Bus Selector3/1 -> Motor On Data Type Conversion1/1  "<rotor_velocity>"
  Motor On Data Type Conversion1/1 -> Motor On Rate Transition1/1
  Motor On Rate Transition1/1 -> Rotor Velocity/1
  Motor On Rate Transition2/1 -> Command1/1  "data"
  Motor On Rate Transition4/1 -> Command2/1  "data"
  Bus Selector/2 -> Motor On Rate Transition2/1  "<Motor_T_Lim>"
  Bus Selector/3 -> Motor On Rate Transition4/1  "<Regen_T_Lim>"

== system EVdemo_6/Drive & Motor/System_Motor/Control_Velocity (Explicit_Ts) ==
  note: Velocity Controller
  note: This simplified controller regulates motor velocity using rotor velocity feedback compared to a commanded velocity.
      | The output of the controller is a power limited torque reference to an idealized drive and motor model.
  velocity_command : Inport
      settings: AttributesFormatString=-----------------------------\nMin = %<OutMin>\nMax = %<OutMax>
  mtr_torque_lim : Inport  Port=2  OutMin=-ctrlConst.VelocityMax  OutMax=ctrlConst.VelocityMax
  regen_torque_lim : Inport  Port=3  OutMin=-ctrlConst.VelocityMax  OutMax=ctrlConst.VelocityMax
  velocity_measured : Inport  Port=4
      settings: AttributesFormatString=-----------------------------\nMin = %<OutMin>\nMax = %<OutMax>
  Error Sum : Sum  Inputs=+-|  OutMin=-2*ctrlConst.VelocityMax  OutMax=2*ctrlConst.VelocityMax  OutDataTypeStr=DT_PRECISION_LO
      settings: AttributesFormatString=-----------------------------\nMin = %<OutMin>\nMax = %<OutMax>
  Rotor_Velocity_Control : Subsystem
      mask Display:
      | disp('PI(z)')
      | port_label('input',1, '');
      | port_label('output',1, '');
  torque_cmd : Outport  InitialOutput=0
  wires:
  velocity_command/1 -> Error Sum/1
  Rotor_Velocity_Control/1(Out) -> torque_cmd/1  "torque_cmd"
  Error Sum/1 -> Rotor_Velocity_Control/1(Err)  "velocity_error"
  velocity_measured/1 -> Error Sum/2
  mtr_torque_lim/1 -> Rotor_Velocity_Control/2(mtr_torque_lim)
  regen_torque_lim/1 -> Rotor_Velocity_Control/3(regen_torque_lim)

== system EVdemo_6/Drive & Motor/System_Motor/Discrete To Continuous1 ==
  note: Discrete To Continuous
  T : Inport
  Motor On Data Type Conversion1 : DataTypeConversion
  Motor On Rate Transition1 : RateTransition  Integrity=off  Deterministic=off
  Motor Command : Outport
  wires:
  T/1 -> Motor On Data Type Conversion1/1
  Motor On Data Type Conversion1/1 -> Motor On Rate Transition1/1
  Motor On Rate Transition1/1 -> Motor Command/1
